simulink model "simple"  (Simulink 3.00)
settings: Solver=ode45  StartTime=0.0  StopTime=10.0  RelTol=1e-3
settings Model: LastModifiedBy=pdm104

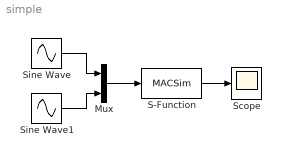
== system simple ==
  Mux : Mux  Inputs=2
  S-Function : S-Function  FunctionName=MACSim  PortCounts=[]  SFunctionModules=''
  Scope : Scope
      settings: TimeRange=auto  YMin=-5  YMax=5  SaveToWorkspace=off  SaveName=ScopeData
  Sine Wave : Sin  Amplitude=1  Frequency=1  Phase=0  SampleTime=0
  Sine Wave1 : Sin  Amplitude=1  Frequency=4  Phase=0  SampleTime=0
  wires:
  Mux/1 -> S-Function/1
  Sine Wave1/1 -> Mux/2
  Sine Wave/1 -> Mux/1
  S-Function/1 -> Scope/1
